simulink model "Tester"  (R2016a)
settings: Solver=VariableStepAuto  StartTime=0.0  StopTime=10.0  RelTol=1e-3
settings Model: Creator=levi.hubbard  LastModifiedBy=levi.hubbard

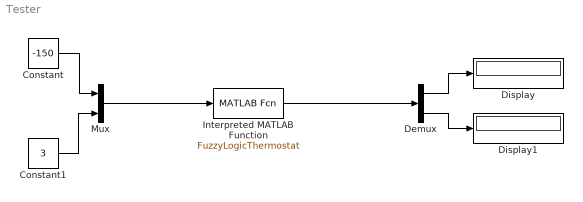
== system Tester ==
  Constant : Constant  Value=-150
  Constant1 : Constant  Value=3
  Demux : Demux  Outputs=2
  Display : Display
  Display1 : Display
  Interpreted MATLAB Function : MATLABFcn  MATLABFcn=FuzzyLogicThermostat
  Mux : Mux  Inputs=2
  wires:
  Mux/1 -> Interpreted MATLAB Function/1
  Constant1/1 -> Mux/2
  Constant/1 -> Mux/1
  Interpreted MATLAB Function/1 -> Demux/1
  Demux/1 -> Display/1
  Demux/2 -> Display1/1
